simulink model "Falling_SRA"  (R2022a)
settings: Solver=VariableStepAuto  StartTime=0.0  StopTime=10.0  RelTol=1e-3
settings Model: Creator=yalun  LastModifiedBy=yalun
settings RTWCC: GenCodeOnly=on

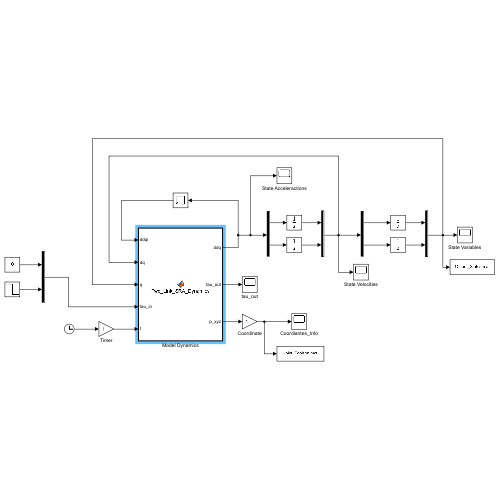
[thumbnail: Simulink's stored preview of the top-level diagram]
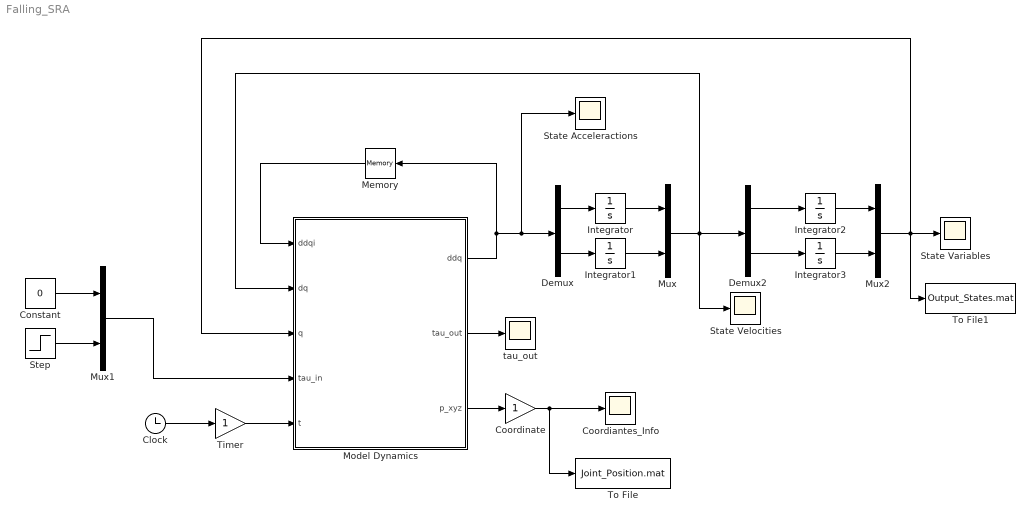
== system Falling_SRA ==
  Clock : Clock
  Constant : Constant  Value=0
  Coordiantes_Info : Scope
  Coordinate : Gain
  Demux : Demux  Outputs=2
  Demux2 : Demux  Outputs=2
  Integrator{,1..3} (4 alike) : Integrator
  Memory : Memory
  Model Dynamics : MATLAB Function  TreatAsAtomicUnit=on
  Mux : Mux  Inputs=2
  Mux1 : Mux  Inputs=2
  Mux2 : Mux  Inputs=2
  State Acceleractions : Scope
  State Variables : Scope
  State Velocities : Scope
  Step : Step  Before=0.03  After=0  SampleTime=0
  Timer : Gain
  To File : ToFile  Filename=Joint_Position.mat  SaveFormat=Timeseries
  To File1 : ToFile  Filename=Output_States.mat  SaveFormat=Timeseries
  tau_out : Scope
  wires:
  Timer/1 -> Model Dynamics/5(t)
  Clock/1 -> Timer/1
  Model Dynamics/1(ddq) -> State Acceleractions/1, Demux/1, Memory/1
  Memory/1 -> Model Dynamics/1(ddqi)
  Model Dynamics/2(tau_out) -> tau_out/1
  Model Dynamics/3(p_xyz) -> Coordinate/1
  Coordinate/1 -> To File/1, Coordiantes_Info/1
  Integrator/1 -> Mux/1
  Integrator1/1 -> Mux/2
  Demux/1 -> Integrator/1
  Demux/2 -> Integrator1/1
  Mux/1 -> State Velocities/1, Model Dynamics/2(dq), Demux2/1
  Demux2/1 -> Integrator2/1
  Integrator3/1 -> Mux2/2
  Demux2/2 -> Integrator3/1
  Integrator2/1 -> Mux2/1
  Mux2/1 -> To File1/1, Model Dynamics/3(q), State Variables/1
  Mux1/1 -> Model Dynamics/4(tau_in)
  Constant/1 -> Mux1/1
  Step/1 -> Mux1/2

== matlab function Falling_SRA/Model Dynamics ==
  data: ddqi input size=2; ddq output size=2; tau_out output size=2; dq input size=2; q input size=2; tau_in input size=2; t input size=1; p_xyz output size=4
function [ddq,tau_out,p_xyz] = Two_Link_SRA_Dynamics(ddqi,dq,q,tau_in,t)

% Similar to C or C++, we have to claim the function we are going to use
% externally.
coder.extrinsic('sym');
coder.extrinsic('symfun');
coder.extrinsic('jacobian');
coder.extrinsic('diff');
coder.extrinsic('subs');
coder.extrinsic('double');


% Fixed position in inertia frame
pfx=-1;
pfy=1;

% The number of link for each side of the SRA.
n_link=2;
ddq=zeros(n_link,1);
tau_out=zeros(n_link,1);



%% SRA Parameters %%
% Segment stiffness
k=[2.5,2];
% Segment damping coefficient
b=[1,0.9];
% Segment length & mass
L=[0.3,0.3];
m=[1.25,1.25];

g=9.81;
%% End %%

theta=sym('theta',[1,n_link]);
R=struct('theta',zeros(4,4));
for i=1:n_link
    % The expression of the standand derived transformation/rotation
    % matrix.
    R(i)=struct('theta',zeros(4,4));
    R(i).theta=[cos(theta(i)) sin(theta(i)) 0 2*L(i)*(sin(theta(i)/2)^2)/theta(i);
    -1*sin(theta(i)) cos(theta(i)) 0 L(i)*sin(theta(i))/theta(i);
    0 0 1 0;
    0 0 0 1];
end

% Calculate the intermediate rotation matrix.
R_intm=struct('theta',zeros(4,4));
for j=1:n_link
    if j==1
        R_intm(j).theta=R(1).theta;
    else
        R_intm(j).theta=R_intm(j-1).theta*R(j).theta;
    end
end

% Twist matrix in 2D problem
% As the SRA was initally horizontally fixed on the wall, it will bounce up
% and down, however, its direction cannot be justified by the theta value
% of SRA, we have to set up an individual transformation matrix rotating around z axis for it.

% 1. Bounce down                                                                                                                                                                                                                                                                                                                                                                                                                                                                                                                                                                                                                                                                                                                                                                                                                                                                                                                                                                                                                                                                                                                                                                                                                                                                                                                                                                                                                                                                                                                                                                                                                                                                                                                                                                                                                                                                                                                                        
Rz_down=[cos(-pi/2) -sin(-pi/2) 0 pfx;
    sin(-pi/2) cos(-pi/2) 0 pfy;
    0 0 1 0;
    0 0 0 1];

% Calculate the energy for each part
% Potential energy due to gravity (the zero potential surface is the vertical position fixed)
p_x=struct('theta',zeros(1,1)); p_y=struct('theta',zeros(1,1));
delta_p_x=struct('theta',zeros(1,1)); delta_p_y=struct('theta',zeros(1,1));
potential_g_y=struct('theta',zeros(1,1));
R_pos=struct('theta',zeros(4,4));
for i=1:n_link
    R_pos(i).theta=Rz_down*R_intm(i).theta;
    p_x(i).theta=R_pos(i).theta(1,4);
    p_y(i).theta=R_pos(i).theta(2,4);
end
for i=1:n_link
    if i==1
        delta_p_y(1).theta=p_x(1).theta-pfx;
        delta_p_x(1).theta=p_y(1).theta-pfy;
    else
        delta_p_y(i).theta=p_x(i).theta-p_x(i-1).theta;
        delta_p_x(i).theta=p_y(i).theta-p_y(i-1).theta;
    end
end
% Calculate the absolute distance between the original inertia frame and
% the COM of each link.
for i=1:n_link
    if i==1
        potential_g_y(1).theta=delta_p_y(1).theta/2;
    else
        % 2022.10.09
        % Still haven't figured out the reason for index expression out of
        % bounds.
        potential_g_y(i).theta=p_y(i-1).theta+delta_p_y(i).theta/2;
    end
end

% Calculate the manipulator Jacobian matrix
o=struct('theta',zeros(3,1)); z=struct('theta',zeros(3,1));
o(1).theta=[pfx;pfy;0];
z(1).theta=[0;0;1];
for i=1:n_link
    o(i+1).theta=[p_x(1).theta;p_y(1).theta;0];
    z(i+1).theta=[R_pos(i).theta(1,3);R_pos(i).theta(2,3);R_pos(i).theta(3,3)];
end
J_v=struct('theta',zeros(3,1)); J_w=struct('theta',zeros(3,1));
for i=1:n_link
    J_v(i).theta=cross(z(i).theta,o(end).theta-o(i).theta);
    J_w(i).theta=z(i).theta;
end

% Kinetic Energy Calculation

% Potential Energy Calculation, which is based on the Lagrange's Equation.
% We don't have to work out the part due to stiffness and damping as they
% are about theta and theta dot respectively.
P_g_real=0;
P_g=struct('theta',zeros(1,1));
for i=1:n_link
    P_g_real=P_g_real+m(i)*g*potential_g_y(i).theta;
end
for i=1:n_link
    P_g(i).theta=diff(P_g_real,theta(i));
end

% Intertia Matrix
J_linear=struct('theta',zeros(2,n_link));
M_linear=struct('theta',zeros(n_link,n_link));
M_angular=struct('theta',zeros(n_link,n_link));
M_total=struct('theta',zeros(n_link,n_link));
I=zeros(n_link,1);
for i=1:n_link
    J_linear(i).theta=jacobian([R_pos(i).theta(1,4),R_pos(i).theta(2,4)],theta);
    M_linear(i).theta=m(i)*transpose(J_linear(i).theta)*J_linear(i).theta;
    I(i)=1/12*m(i)*(L(i))^2;
    J_angular=zeros(1,n_link);
    J_angular(1:i)=1;
    M_angular(i).theta=I(i)*1/2*transpose(J_angular)*1/2*J_angular;
    M_total(i).theta=M_linear(i).theta+M_angular(i).theta;
end
M=zeros(n_link,n_link);
for i=1:n_link
    M=M+M_total(i).theta;
end

% Centripetal-Coriolis Matrix

theta_dot=sym('theta_dot',[1,n_link]);
sum_element=0;
sum_intm=struct('theta',zeros(1,1));
C_element=struct('theta',zeros(n_link,n_link));
c1=struct('theta',zeros(1,1));
c2=struct('theta',zeros(1,1));
c3=struct('theta',zeros(1,1));

% 2022.10.09
% Bad example of cell use, although in this step, there is no warning or
% error indication that it's not available to use cell definition and
% establishment. All terms containing symbolic variables should be stored
% in struct, and for external function in MATLAB, Simulink can only cope
% with one of them at one time, so we should write them separately.
% for i=1:n_link
%     for j=1:n_link
%         C_element{i,j}=0;
%     end
% end

for i=1:n_link
    for j=1:n_link
        for k=1:n_link
            c1(i,j).theta=diff(M(i,j),theta(k));
            c2(i,j).theta=diff(M(i,k),theta(j));
            c3(i,j).theta=diff(M(k,j),theta(i));
            sum_intm(i,j).theta=1/2*(c1(i,j).theta+c2(i,j).theta-c3(i,j).theta)*theta_dot(k);
%             sum_intm(i).theta=1/2*(diff(M(k,j),theta(j))+diff(M(k,i),theta(j))-diff(M(i,j),theta(k)))*theta_dot(i);
            sum_element=sum_element+sum_intm(i,j).theta;
        end
        C_element.theta(i,j)=sum_element;
    end
end



%% Reprocessing the matrix above %%

M=double(subs(M,theta,transpose(q)));
C_element.theta=double(subs(C_element.theta,[theta,theta_dot],[transpose(q),transpose(dq)]));
% R.theta=double(subs(R.theta,theta,q)); R_intm.theta=double(subs(R_intm.theta,theta,q)); R_pos.theta=double(subs(R_pos.theta,theta,q));
p_x.theta=double(subs(p_x.theta,theta,transpose(q)));
p_y.theta=double(subs(p_y.theta,theta,transpose(q)));
% Concert the cell format into matrix format for matrix computation.
C=zeros(n_link,n_link);
for i=n_link
    for j=1:n_link
        C(i,j)=double(C_element.theta(i,j));
    end
end
Pg=zeros(n_link,1); Pk=zeros(n_link,1); Pb=zeros(n_link,1);
for i=1:n_link
    P_g(i).theta=double(subs(P_g(i).theta,theta,transpose(q)));
    Pg(i,1)=P_g(i).theta;
    Pk(i,1)=double(k(i)*q(i));
    Pb(i,1)=double(b(i)*dq(i));
end

%% Test Code %%
% 2022.10.10
% M=[6 3; 3 6];
% C=[4 3; 8 6];
% Pg=[1;1];
%% End %%

ddq=double(M\(tau_in-C*dq-Pg-Pk-Pb));
tau_out=double(M*ddqi+C*dq+Pg+Pk+Pb);
p_xyz=zeros(2*n_link,1);
for i=1:n_link
    p_xyz(2*i-1)=p_x(i).theta;
    p_xyz(2*i)=p_y(i).theta;
end
p_xyz=double(p_xyz);
end
